simulink model "q_heli_2d_ff_lqr_i"  (Simulink 7.7)
settings: Solver=ode1  StartTime=0.0  StopTime=inf  FixedStep=0.002  MaxStep=10  RelTol=1e-3  AbsTol=1e-3
values from neighbouring files (symbols this model uses):
  g = 9.81    [setup_heli_2d_configuration.m]
  INT_JOYSTICK_SAT_LOWER = theta_0 * 180 / pi    (= -40.5)    [setup_lab_heli_2d.m]
  INT_JOYSTICK_SAT_UPPER = abs(theta_0)  * 180 / pi    [setup_lab_heli_2d.m]
  J_eq_p = J_m_p + J_body_p + J_p + J_y    (= 0.0384309870395)    [setup_heli_2d_configuration.m]
  J_eq_y = J_m_y + J_body_y + J_p + J_y + J_shaft    (= 0.0431517259335)    [setup_heli_2d_configuration.m]
  JOYSTICK_X_DZ = 0.25    [setup_lab_heli_2d.m]
  JOYSTICK_Y_DZ = 0.25    [setup_lab_heli_2d.m]
  K_AMP = 3    [setup_lab_heli_2d.m]
  K_EC_P = - 2 * pi / ( 4 * 1024 )    (= -0.00153398078789)    [setup_lab_heli_2d.m]
  K_EC_Y = 2 * pi / ( 8 * 1024 )    (= 0.000766990393943)    [setup_lab_heli_2d.m]
  K_ff = 1    [setup_lab_heli_2d.m]
  K_JOYSTICK_X = 85    [setup_lab_heli_2d.m]
  K_JOYSTICK_Y = 85    [setup_lab_heli_2d.m]
  K_pp = K_f_p * r_p    (= 0.20413345)    [setup_heli_2d_configuration.m]
  K_py = K_t_y / R_m_y    (= 0.0068125)    [setup_heli_2d_configuration.m]
  K_yp = K_t_p / R_m_p    (= 0.0219277108434)    [setup_heli_2d_configuration.m]
  K_yy = K_f_y * r_y    (= 0.071988045)    [setup_heli_2d_configuration.m]
  l_cm = ( (m_motor_p + m_shield ) * r_p +  (m_motor_y + m_shield ) * r_y ) / ( m_props )    (= 0.185670125995)    [setup_heli_2d_configuration.m]
  m_heli = 1.3872    [setup_heli_2d_configuration.m]
  SAT_INT_ERR_PITCH = 8    [setup_lab_heli_2d.m]
  SAT_INT_ERR_YAW = 8    [setup_lab_heli_2d.m]
  theta_0 = -40.5*pi/180    (= -0.706858347058)    [setup_lab_heli_2d.m]
  Tr_p = 1    [setup_lab_heli_2d.m]
  Tr_y = 1    [setup_lab_heli_2d.m]
  VMAX_AMP_P = 24    [setup_lab_heli_2d.m]
  VMAX_AMP_Y = 15    [setup_lab_heli_2d.m]
  wcf = 2 * pi * 20    (= 125.663706144)    [setup_lab_heli_2d.m]
  zetaf = 0.85    [setup_lab_heli_2d.m]
undefined symbols (not defined in the file or in its folder): B_p, B_y, HIL, K, Ki, qc_get_step_size
libraries: simulink x9, simulink_extras x7, quarc_library x4
settings Model: Creator=MLevis  LastModifiedBy=pmartin  SimulationMode=external  ExtModeTrigDuration=50000  BufferReuse=off
settings SolverCC: PositivePriorityOrder=on
settings DataIOCC: LimitDataPoints=off  SaveOutput=off  SaveTime=off  SignalLoggingName=sigsOut
settings OptimizationCC: BlockReduction=off  BooleanDataType=off  InlineInvariantSignals=on  OptimizeBlockIOStorage=off  BufferReuse=off  ExpressionFolding=off  LocalBlockOutputs=off  InitFltsAndDblsToZero=on
settings DebuggingCC: SaveWithParameterizedLinksMsg=none  SignalResolutionControl=TryResolveAllWithWarning  SolverPrmCheckMsg=none  MultiTaskDSMMsg=warning  MultiTaskCondExecSysMsg=none  StrictBusMsg=None
settings RTWCC: SystemTargetFile=quarc_windows.tlc  TemplateMakefile=quarc_default_tmf  Description=QuaRC Win32 Target  ProcessScript=quarc_windows_make_rtw_hook  IncludeERTFirstTime=on
settings STFCustomTargetCC: TargetFcnLib=ansi_tfl_tmw.mat  TargetPreCompLibLocation=C:\PROGRA~3\QUARC\lib\2012b\windows\release  GeneratePreprocessorConditionals=Disable all  SystemTargetFile=quarc_windows.tlc
settings GRTTargetCC: TargetFcnLib=ansi_tfl_tmw.mat  TargetPreCompLibLocation=C:\PROGRA~3\QUARC\lib\2012b\windows\release  ParMdlRefBuildCompliant=off  CompOptLevelCompliant=off  MatFileLogging=off  ExtMode=on  ExtModeMexFile=quarc_comm

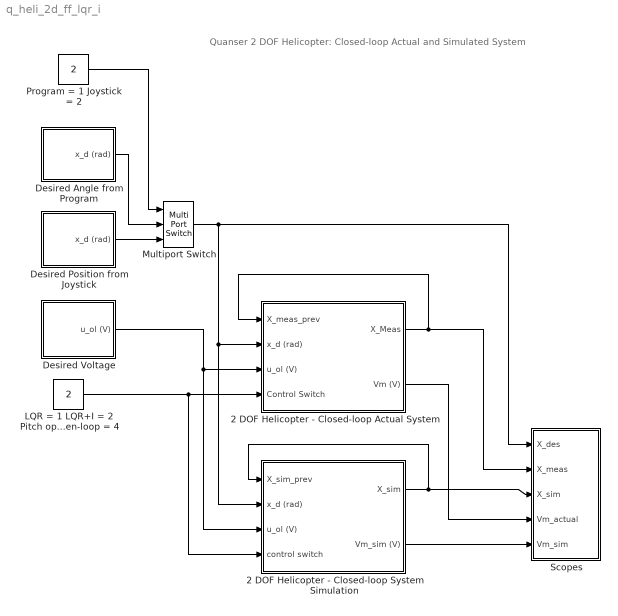
== system q_heli_2d_ff_lqr_i ==
  note: Quanser 2 DOF Helicopter:
      | Closed-loop Actual and Simulated System
  2 DOF Helicopter - Closed-loop Actual System : Subsystem
  2 DOF Helicopter - Closed-loop System Simulation : Subsystem
  Desired Angle from Program : Subsystem
  Desired Position from Joystick : Subsystem
  Desired Voltage : Subsystem
  LQR = 1 LQR+I = 2 Pitch open-loop  = 3 Yaw open-loop = 4 : Constant  Value=2
  Multiport Switch : MultiPortSwitch  Inputs=2
  Program = 1 Joystick = 2 : Constant  Value=2
  Scopes : Subsystem
  wires:
  2 DOF Helicopter - Closed-loop System Simulation/1(X_sim) -> Scopes/3(X_sim), 2 DOF Helicopter - Closed-loop System Simulation/1(X_sim_prev)
  2 DOF Helicopter - Closed-loop Actual System/1(X_Meas) -> Scopes/2(X_meas), 2 DOF Helicopter - Closed-loop Actual System/1(X_meas_prev)
  2 DOF Helicopter - Closed-loop Actual System/2(Vm (V)) -> Scopes/4(Vm_actual)
  LQR = 1 LQR+I = 2 Pitch open-loop  = 3 Yaw open-loop = 4/1 -> 2 DOF Helicopter - Closed-loop Actual System/4(Control Switch), 2 DOF Helicopter - Closed-loop System Simulation/4(control switch)
  2 DOF Helicopter - Closed-loop System Simulation/2(Vm_sim (V)) -> Scopes/5(Vm_sim)
  Desired Voltage/1(u_ol (V)) -> 2 DOF Helicopter - Closed-loop Actual System/3(u_ol (V)), 2 DOF Helicopter - Closed-loop System Simulation/3(u_ol (V))
  Program = 1 Joystick = 2/1 -> Multiport Switch/1
  Desired Angle from Program/1(x_d (rad)) -> Multiport Switch/2
  Desired Position from Joystick/1(x_d (rad)) -> Multiport Switch/3
  Multiport Switch/1 -> Scopes/1(X_des), 2 DOF Helicopter - Closed-loop Actual System/2(x_d (rad)), 2 DOF Helicopter - Closed-loop System Simulation/2(x_d (rad))

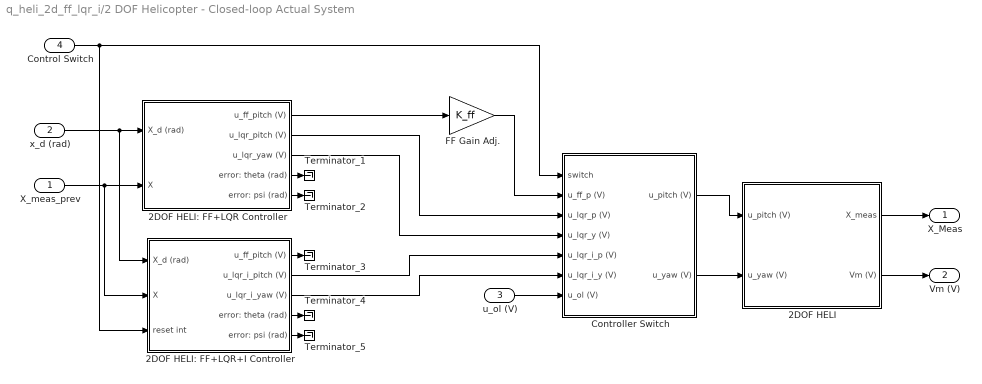
== system q_heli_2d_ff_lqr_i/2 DOF Helicopter - Closed-loop Actual System ==
  X_meas_prev : Inport
  x_d (rad) : Inport  Port=2
  u_ol (V) : Inport  Port=3
  Control Switch : Inport  Port=4
  2DOF HELI : Subsystem
  2DOF HELI: FF+LQR Controller : Subsystem
  2DOF HELI: FF+LQR+I Controller : Subsystem
  Controller Switch : Subsystem
  FF Gain Adj. : Gain  Gain=K_ff
  Terminator_{1..5} (5 alike) : Terminator
  X_Meas : Outport
  Vm (V) : Outport  Port=2
  wires:
  2DOF HELI: FF+LQR+I Controller/5(error: psi (rad)) -> Terminator_5/1
  2DOF HELI: FF+LQR+I Controller/4(error: theta (rad)) -> Terminator_4/1
  2DOF HELI: FF+LQR+I Controller/1(u_ff_pitch (V)) -> Terminator_3/1
  2DOF HELI: FF+LQR Controller/5(error: psi (rad)) -> Terminator_2/1
  2DOF HELI: FF+LQR Controller/4(error: theta (rad)) -> Terminator_1/1
  u_ol (V)/1 -> Controller Switch/7(u_ol (V))
  2DOF HELI: FF+LQR+I Controller/3(u_lqr_i_yaw (V)) -> Controller Switch/6(u_lqr_i_y (V))
  2DOF HELI: FF+LQR+I Controller/2(u_lqr_i_pitch (V)) -> Controller Switch/5(u_lqr_i_p (V))
  Controller Switch/2(u_yaw (V)) -> 2DOF HELI/2(u_yaw (V))
  Controller Switch/1(u_pitch (V)) -> 2DOF HELI/1(u_pitch (V))
  2DOF HELI: FF+LQR Controller/2(u_lqr_pitch (V)) -> Controller Switch/3(u_lqr_p (V))
  FF Gain Adj./1 -> Controller Switch/2(u_ff_p (V))
  2DOF HELI: FF+LQR Controller/3(u_lqr_yaw (V)) -> Controller Switch/4(u_lqr_y (V))
  X_meas_prev/1 -> 2DOF HELI: FF+LQR+I Controller/2(X), 2DOF HELI: FF+LQR Controller/2(X)
  x_d (rad)/1 -> 2DOF HELI: FF+LQR+I Controller/1(X_d (rad)), 2DOF HELI: FF+LQR Controller/1(X_d (rad))
  2DOF HELI: FF+LQR Controller/1(u_ff_pitch (V)) -> FF Gain Adj./1
  Control Switch/1 -> Controller Switch/1(switch), 2DOF HELI: FF+LQR+I Controller/3(reset int)
  2DOF HELI/2(Vm (V)) -> Vm (V)/1
  2DOF HELI/1(X_meas) -> X_Meas/1

== system q_heli_2d_ff_lqr_i/2 DOF Helicopter - Closed-loop System Simulation ==
  X_sim_prev : Inport
  x_d (rad) : Inport  Port=2
  u_ol (V) : Inport  Port=3
  control switch : Inport  Port=4
  2DOF HELI: FF+LQR Controller : Subsystem
  2DOF HELI: FF+LQR+I Controller : Subsystem
  2DOF HELI: Nonlinear Model : Subsystem
  Controller Switch : Subsystem
  Terminator_{1..5} (5 alike) : Terminator
  X_sim : Outport
  Vm_sim (V) : Outport  Port=2
  wires:
  2DOF HELI: FF+LQR+I Controller/5(error: psi (rad)) -> Terminator_5/1
  2DOF HELI: FF+LQR+I Controller/4(error: theta (rad)) -> Terminator_4/1
  2DOF HELI: FF+LQR+I Controller/1(u_ff_pitch (V)) -> Terminator_3/1
  2DOF HELI: FF+LQR Controller/5(error: psi (rad)) -> Terminator_2/1
  2DOF HELI: FF+LQR Controller/4(error: theta (rad)) -> Terminator_1/1
  u_ol (V)/1 -> Controller Switch/7(u_ol (V))
  2DOF HELI: Nonlinear Model/1(X_sim) -> X_sim/1
  2DOF HELI: Nonlinear Model/2(V_m_sim (V)) -> Vm_sim (V)/1
  control switch/1 -> 2DOF HELI: FF+LQR+I Controller/3(reset int), Controller Switch/1(switch)
  2DOF HELI: FF+LQR+I Controller/2(u_lqr_i_pitch (V)) -> Controller Switch/5(u_lqr_i_p (V))
  2DOF HELI: FF+LQR Controller/3(u_lqr_yaw (V)) -> Controller Switch/4(u_lqr_y (V))
  2DOF HELI: FF+LQR Controller/1(u_ff_pitch (V)) -> Controller Switch/2(u_ff_p (V))
  2DOF HELI: FF+LQR Controller/2(u_lqr_pitch (V)) -> Controller Switch/3(u_lqr_p (V))
  2DOF HELI: FF+LQR+I Controller/3(u_lqr_i_yaw (V)) -> Controller Switch/6(u_lqr_i_y (V))
  X_sim_prev/1 -> 2DOF HELI: FF+LQR+I Controller/2(X), 2DOF HELI: FF+LQR Controller/2(X)
  x_d (rad)/1 -> 2DOF HELI: FF+LQR Controller/1(X_d (rad)), 2DOF HELI: FF+LQR+I Controller/1(X_d (rad))
  Controller Switch/1(u_pitch (V)) -> 2DOF HELI: Nonlinear Model/1(u_pitch (V))
  Controller Switch/2(u_yaw (V)) -> 2DOF HELI: Nonlinear Model/2(u_yaw (V))

== system q_heli_2d_ff_lqr_i/Desired Angle from Program ==
  note: Desired yaw angle
  note: Desired pitch angle
  Amplitude: Pitch (deg) : Gain  Gain=0
  Amplitude: Yaw (deg) : Gain  Gain=0
  Constant : Constant
  Constant: Pitch (deg) : simulink/Math Operations/Slider Gain  low=-30  gain=-30  high=15
  Constant: Yaw (deg) : Constant  Value=0
  Mux : Mux  Inputs=2
  Pitch: deg to rad : simulink_extras/Transformations/Degrees to Radians
  Signal Generator: Pitch : SignalGenerator  WaveForm=square  Frequency=0.05
  Signal Generator: Yaw : SignalGenerator  WaveForm=square  Frequency=0.05
  Sum : Sum  Inputs=|++
  Sum1 : Sum  Inputs=|++
  Yaw: deg to rad : simulink_extras/Transformations/Degrees to Radians
  x_d (rad) : Outport
  wires:
  Constant: Pitch (deg)/1 -> Sum/2
  Yaw: deg to rad/1 -> Mux/2
  Mux/1 -> x_d (rad)/1
  Constant: Yaw (deg)/1 -> Sum1/2
  Amplitude: Yaw (deg)/1 -> Sum1/1
  Signal Generator: Yaw/1 -> Amplitude: Yaw (deg)/1
  Sum1/1 -> Yaw: deg to rad/1
  Constant/1 -> Constant: Pitch (deg)/1
  Amplitude: Pitch (deg)/1 -> Sum/1
  Signal Generator: Pitch/1 -> Amplitude: Pitch (deg)/1
  Sum/1 -> Pitch: deg to rad/1
  Pitch: deg to rad/1 -> Mux/1

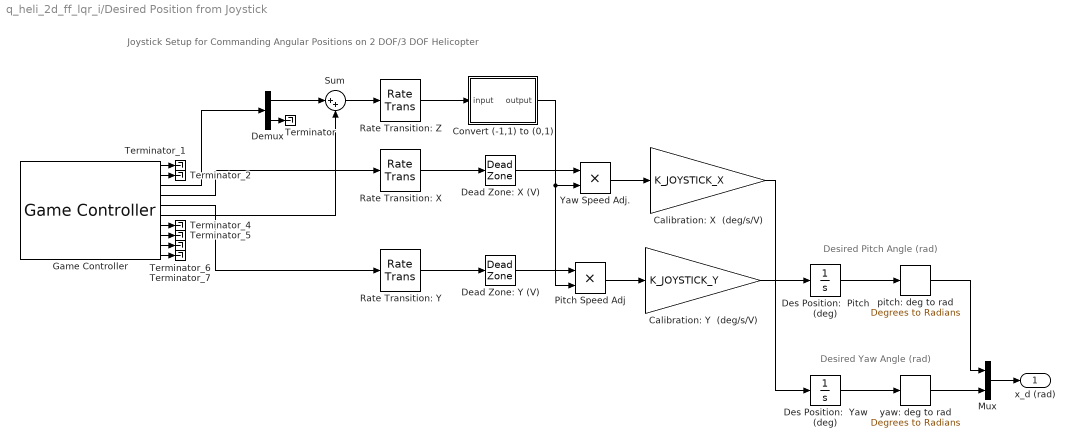
== system q_heli_2d_ff_lqr_i/Desired Position from Joystick ==
  note: Desired Pitch Angle (rad)
  note: Desired Yaw Angle (rad)
  note: Joystick Setup for Commanding Angular Positions on 2 DOF/3 DOF Helicopter
  Calibration: X  (deg/s/V) : Gain  Gain=K_JOYSTICK_X
  Calibration: Y  (deg/s/V) : Gain  Gain=K_JOYSTICK_Y
  Convert (-1,1) to (0,1) : Subsystem
  Dead Zone: X (V) : DeadZone  LowerValue=-JOYSTICK_X_DZ  UpperValue=JOYSTICK_X_DZ  SaturateOnIntegerOverflow=on
  Dead Zone: Y (V) : DeadZone  LowerValue=-JOYSTICK_Y_DZ  UpperValue=JOYSTICK_Y_DZ  SaturateOnIntegerOverflow=on
  Demux : Demux  Outputs=2
  Des Position:  Pitch (deg) : Integrator  InitialCondition=theta_0*180/pi  LimitOutput=on  UpperSaturationLimit=INT_JOYSTICK_SAT_UPPER  LowerSaturationLimit=INT_JOYSTICK_SAT_LOWER
  Des Position:  Yaw (deg) : Integrator  UpperSaturationLimit=180  LowerSaturationLimit=-180
  Game Controller : quarc_library/Devices/Peripherals/Target/Game Controller  controller=1  buffer_size=12  deadzone=[]  saturation=[]  sample_time=max(qc_get_step_size, 0.01)  auto_center=off  enabled=on
  Mux : Mux  Inputs=2
  Pitch Speed Adj : Product  RndMeth=Zero
  Rate Transition: X : RateTransition
  Rate Transition: Y : RateTransition
  Rate Transition: Z : RateTransition
  Sum : Sum  Inputs=|++
  Terminator : Terminator
  Terminator_{1..2,4..7} (6 alike) : Terminator
  Yaw Speed Adj. : Product  RndMeth=Zero
  pitch: deg to rad : simulink_extras/Transformations/Degrees to Radians
  yaw: deg to rad : simulink_extras/Transformations/Degrees to Radians
  x_d (rad) : Outport
  wires:
  Des Position:  Pitch (deg)/1 -> pitch: deg to rad/1
  Des Position:  Yaw (deg)/1 -> yaw: deg to rad/1
  Mux/1 -> x_d (rad)/1
  Calibration: X  (deg/s/V)/1 -> Des Position:  Yaw (deg)/1
  Dead Zone: X (V)/1 -> Yaw Speed Adj./1
  Dead Zone: Y (V)/1 -> Pitch Speed Adj/1
  pitch: deg to rad/1 -> Mux/1
  yaw: deg to rad/1 -> Mux/2
  Yaw Speed Adj./1 -> Calibration: X  (deg/s/V)/1
  Pitch Speed Adj/1 -> Calibration: Y  (deg/s/V)/1
  Calibration: Y  (deg/s/V)/1 -> Des Position:  Pitch (deg)/1
  Convert (-1,1) to (0,1)/1(output) -> Yaw Speed Adj./2, Pitch Speed Adj/2
  Rate Transition: X/1 -> Dead Zone: X (V)/1
  Rate Transition: Y/1 -> Dead Zone: Y (V)/1
  Rate Transition: Z/1 -> Convert (-1,1) to (0,1)/1(input)
  Game Controller/4 -> Rate Transition: X/1
  Game Controller/5 -> Rate Transition: Y/1
  Game Controller/1 -> Terminator_1/1
  Game Controller/2 -> Terminator_2/1
  Game Controller/7 -> Terminator_4/1
  Game Controller/8 -> Terminator_5/1
  Game Controller/9 -> Terminator_6/1
  Game Controller/10 -> Terminator_7/1
  Sum/1 -> Rate Transition: Z/1
  Game Controller/6 -> Sum/2
  Game Controller/3 -> Demux/1
  Demux/1 -> Sum/1
  Demux/2 -> Terminator/1

== system q_heli_2d_ff_lqr_i/Desired Voltage ==
  note: Desired pitch open-loop voltage
  note: Desired yaw open-loop voltage
  Amplitude: Pitch (V) : Gain  Gain=0.2
  Amplitude: Yaw (V) : Gain  Gain=2.5
  Constant: Pitch (V) : Constant  Value=0
  Constant: Yaw (V) : Constant  Value=0
  Mux : Mux  Inputs=2
  Signal Generator: Pitch (V) : SignalGenerator  WaveForm=square  Frequency=0.4
  Signal Generator: Yaw (V) : SignalGenerator  WaveForm=square  Frequency=0.01
  Sum : Sum  Inputs=|++
  Sum1 : Sum  Inputs=|++
  u_ol (V) : Outport
  wires:
  Constant: Pitch (V)/1 -> Sum/2
  Amplitude: Pitch (V)/1 -> Sum/1
  Signal Generator: Pitch (V)/1 -> Amplitude: Pitch (V)/1
  Constant: Yaw (V)/1 -> Sum1/2
  Amplitude: Yaw (V)/1 -> Sum1/1
  Signal Generator: Yaw (V)/1 -> Amplitude: Yaw (V)/1
  Sum/1 -> Mux/1
  Sum1/1 -> Mux/2
  Mux/1 -> u_ol (V)/1

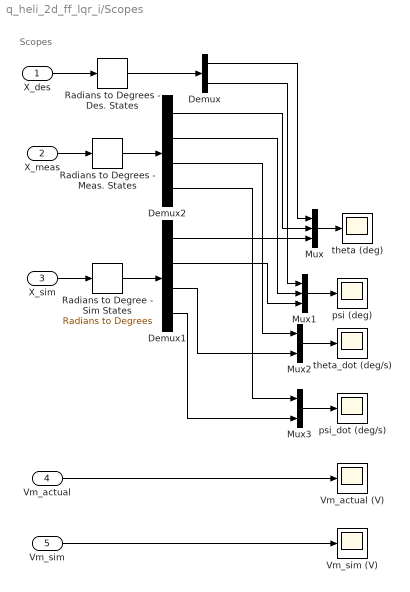
== system q_heli_2d_ff_lqr_i/Scopes ==
  note: Scopes
  X_des : Inport
  X_meas : Inport  Port=2
  X_sim : Inport  Port=3
  Vm_actual : Inport  Port=4
  Vm_sim : Inport  Port=5
  Demux : Demux  Outputs=2
  Demux1 : Demux
  Demux2 : Demux
  Mux : Mux  Inputs=3
  Mux1 : Mux  Inputs=3
  Mux2 : Mux  Inputs=2
  Mux3 : Mux  Inputs=2
  Radians to Degree - Sim States : simulink_extras/Transformations/Radians to Degrees
  Radians to Degrees - Des. States : simulink_extras/Transformations/Radians to Degrees
  Radians to Degrees - Meas. States : simulink_extras/Transformations/Radians to Degrees
  Vm_actual (V) : Scope
      settings: TickLabels=on  TimeRange=50  YMax=15  SaveName=ScopeData4
  Vm_sim (V) : Scope
      settings: TickLabels=on  TimeRange=1.000000  YMin=-250  YMax=250  SaveName=ScopeData5
  psi (deg) : Scope
      settings: TickLabels=on  TimeRange=50  YMin=-70  YMax=90
  psi_dot (deg/s) : Scope
      settings: TickLabels=on  TimeRange=1.000000  YMin=-250  YMax=250  SaveName=ScopeData3
  theta (deg) : Scope
      settings: TickLabels=on  TimeRange=50  YMin=-27.5  YMax=30
  theta_dot (deg/s) : Scope
      settings: TickLabels=on  TimeRange=1.000000  YMax=3.5  SaveName=ScopeData2
  wires:
  Vm_sim/1 -> Vm_sim (V)/1
  Radians to Degrees - Des. States/1 -> Demux/1
  Demux1/2 -> Mux1/3
  Demux2/2 -> Mux1/2
  Demux/2 -> Mux1/1
  Demux1/1 -> Mux/3
  Demux2/1 -> Mux/2
  Demux/1 -> Mux/1
  X_des/1 -> Radians to Degrees - Des. States/1
  Demux2/3 -> Mux2/1
  Demux2/4 -> Mux3/1
  X_meas/1 -> Radians to Degrees - Meas. States/1
  Radians to Degrees - Meas. States/1 -> Demux2/1
  X_sim/1 -> Radians to Degree - Sim States/1
  Radians to Degree - Sim States/1 -> Demux1/1
  Mux/1 -> theta (deg)/1
  Mux1/1 -> psi (deg)/1
  Mux2/1 -> theta_dot (deg/s)/1
  Mux3/1 -> psi_dot (deg/s)/1
  Demux1/3 -> Mux2/2
  Demux1/4 -> Mux3/2
  Vm_actual/1 -> Vm_actual (V)/1

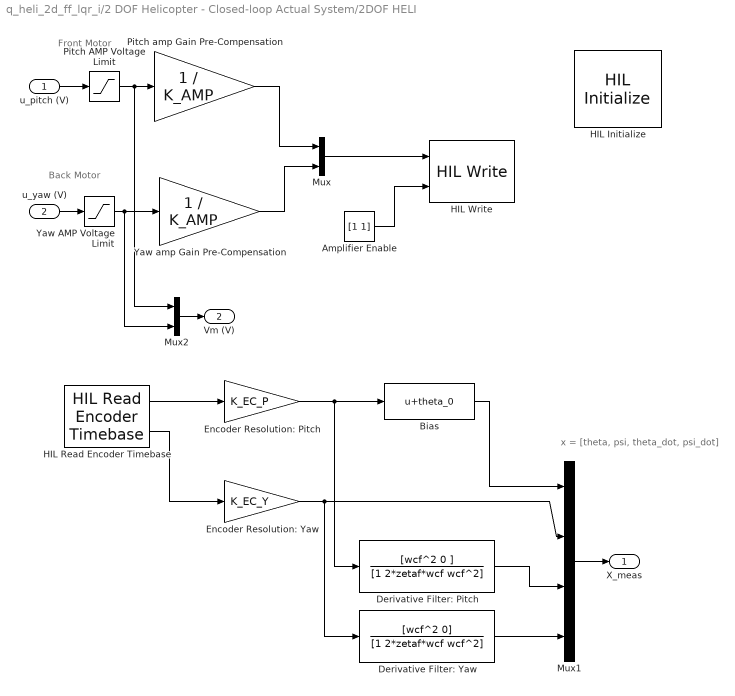
== system q_heli_2d_ff_lqr_i/2 DOF Helicopter - Closed-loop Actual System/2DOF HELI ==
  note: x = [theta, psi, theta_dot, psi_dot]
  note: Front Motor
  note: Back Motor
  u_pitch (V) : Inport
  u_yaw (V) : Inport  Port=2
  Amplifier Enable : Constant  Value=[1 1]
  Bias : Bias  Bias=theta_0
  Derivative Filter: Pitch : TransferFcn  Numerator=[wcf^2 0 ]  Denominator=[1 2*zetaf*wcf wcf^2]
  Derivative Filter: Yaw : TransferFcn  Numerator=[wcf^2 0]  Denominator=[1 2*zetaf*wcf wcf^2]
  "Encoder Resolution: Pitch " : Gain  Gain=K_EC_P
  Encoder Resolution: Yaw : Gain  Gain=K_EC_Y
  HIL Initialize : quarc_library/Data Acquisition/Generic/Configuration/HIL Initialize  object_name=HIL-1  board_type=q2_usb  board_number=0  board_options=d0=digital;d1=digital;led=auto;update_rate=normal;decimation=1  exclusive=off  active=on  hardware_clocks=[0]  clock_modes=[]  initial_clock_frequencies=[]  set_clock_params_at_start=off  set_clock_params_at_switch_in=off  set_clock_frequencies_at_start=off  set_clock_frequencies_at_switch_in=off  analog_input_channels=[0:1]  analog_input_maximums=10  analog_input_minimums=-10  set_analog_input_params_at_start=on  set_analog_input_params_at_switch_in=off  analog_output_channels=[0:1]  analog_output_maximums=10  analog_output_minimums=-10  initial_analog_outputs=[0]  final_analog_outputs=[0]  watchdog_analog_outputs=0  set_analog_output_params_at_start=on  set_analog_output_params_at_switch_in=off  set_analog_outputs_at_start=on  set_analog_outputs_at_switch_in=off  set_analog_outputs_at_terminate=on  set_analog_outputs_at_switch_out=off  set_analog_outputs_on_watchdog=off  digital_input_channels=[]  digital_output_channels=[0:1]  digital_output_configuration=[]  initial_digital_outputs=[0]  final_digital_outputs=[0]  watchdog_digital_outputs=[0]  set_digital_output_params_at_start=off  set_digital_output_params_at_switch_in=off  set_digital_outputs_at_start=on  set_digital_outputs_at_switch_in=off  set_digital_outputs_at_terminate=on  set_digital_outputs_at_switch_out=off  set_digital_outputs_on_watchdog=on  encoder_channels=[0:1]  quadrature=[4]  encoder_filter_frequency=[]  initial_encoder_counts=[0]  set_encoder_params_at_start=on  set_encoder_params_at_switch_in=off  set_encoder_counts_at_start=on  set_encoder_counts_at_switch_in=off  pwm_channels=[]  pwm_modes=[0]  pwm_frequency=1/0.020  pwm_configuration=[]  pwm_alignment=[]  pwm_polarity=[]  pwm_leading_deadband=[]  pwm_trailing_deadband=[]  initial_pwm_outputs=[0]  final_pwm_outputs=[0]  watchdog_pwm_outputs=[0]  set_pwm_params_at_start=on  set_pwm_params_at_switch_in=off  set_pwm_outputs_at_start=on  set_pwm_outputs_at_switch_in=off  set_pwm_outputs_at_terminate=on  set_pwm_outputs_at_switch_out=off  set_pwm_outputs_on_watchdog=off  other_output_channels=[]  initial_other_outputs=[]  final_other_outputs=[]  watchdog_other_outputs=[]  set_other_outputs_at_start=off  set_other_outputs_at_switch_in=off  set_other_outputs_at_terminate=off  set_other_outputs_at_switch_out=off  set_other_outputs_on_watchdog=off
  HIL Read Encoder Timebase : quarc_library/Data Acquisition/Generic/Timebases/HIL Read Encoder Timebase  object_name=HIL-1  clock=0  channels=[0:1]  samples_in_buffer=max(ceil(1/qc_get_step_size), 1)  active=on  vector_output=off  data_type_mode=Inherit via back propagation  data_type=double
  HIL Write : quarc_library/Data Acquisition/Generic/Immediate I//O/HIL Write  object_name=HIL-1  analog_channels=0:1  pwm_channels=[]  digital_channels=0:1  other_channels=[]  sample_time=-1  active=off  vector_input=on
  Mux : Mux  Inputs=2
  Mux1 : Mux
  Mux2 : Mux  Inputs=2
  Pitch AMP Voltage Limit : Saturate  UpperLimit=VMAX_AMP_P  LowerLimit=- VMAX_AMP_P
  Pitch amp Gain Pre-Compensation : Gain  Gain=1 / K_AMP  SaturateOnIntegerOverflow=on  OutDataTypeStr=Inherit: Same as input  ParamDataTypeStr=Inherit: Same as input
  Yaw AMP Voltage Limit : Saturate  UpperLimit=VMAX_AMP_Y  LowerLimit=- VMAX_AMP_Y
  Yaw amp Gain Pre-Compensation : Gain  Gain=1 / K_AMP  SaturateOnIntegerOverflow=on  OutDataTypeStr=Inherit: Same as input  ParamDataTypeStr=Inherit: Same as input
  X_meas : Outport
  Vm (V) : Outport  Port=2
  wires:
  Derivative Filter: Yaw/1 -> Mux1/4
  Derivative Filter: Pitch/1 -> Mux1/3
  Bias/1 -> Mux1/1
  HIL Read Encoder Timebase/2 -> Encoder Resolution: Yaw/1
  "Encoder Resolution: Pitch "/1 -> Derivative Filter: Pitch/1, Bias/1
  HIL Read Encoder Timebase/1 -> "Encoder Resolution: Pitch "/1
  Mux/1 -> HIL Write/1
  Pitch AMP Voltage Limit/1 -> Pitch amp Gain Pre-Compensation/1, Mux2/1
  Yaw AMP Voltage Limit/1 -> Yaw amp Gain Pre-Compensation/1, Mux2/2
  u_pitch (V)/1 -> Pitch AMP Voltage Limit/1
  u_yaw (V)/1 -> Yaw AMP Voltage Limit/1
  Mux1/1 -> X_meas/1
  Pitch amp Gain Pre-Compensation/1 -> Mux/1
  Yaw amp Gain Pre-Compensation/1 -> Mux/2
  Mux2/1 -> Vm (V)/1
  Encoder Resolution: Yaw/1 -> Derivative Filter: Yaw/1, Mux1/2
  Amplifier Enable/1 -> HIL Write/2

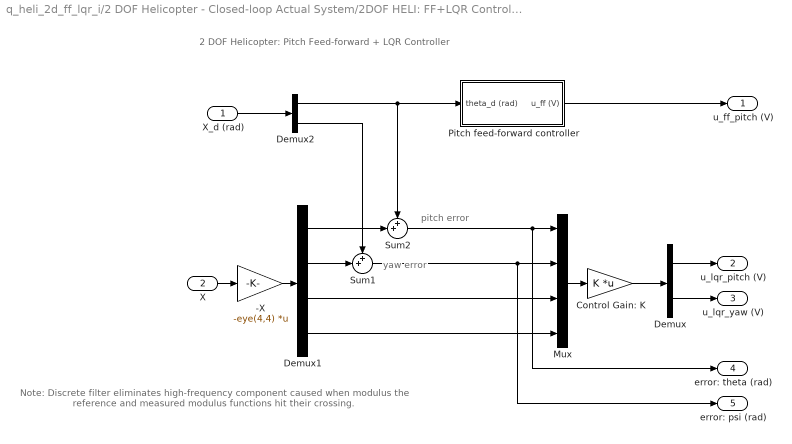
== system q_heli_2d_ff_lqr_i/2 DOF Helicopter - Closed-loop Actual System/2DOF HELI: FF+LQR Controller ==
  note: yaw error
  note: pitch error
  note: 2 DOF Helicopter:
      | Pitch Feed-forward + LQR Controller
  note: Note: Discrete filter eliminates high-frequency
      | component caused when modulus the reference
      | and measured modulus functions hit their crossing.
  X_d (rad) : Inport
  X : Inport  Port=2
  -X : Gain  Gain=-eye(4,4)  Multiplication=Matrix(K*u)
  Control Gain: K : Gain  Gain=K  Multiplication=Matrix(K*u)
  Demux : Demux  Outputs=2
  Demux1 : Demux
  Demux2 : Demux  Outputs=2
  Mux : Mux
  Pitch feed-forward controller : Subsystem
  Sum1 : Sum  Inputs=++|
  Sum2 : Sum  Inputs=++|
  u_ff_pitch (V) : Outport
  u_lqr_pitch (V) : Outport  Port=2
  u_lqr_yaw (V) : Outport  Port=3
  error: theta (rad) : Outport  Port=4
  error: psi (rad) : Outport  Port=5
  wires:
  Pitch feed-forward controller/1(u_ff (V)) -> u_ff_pitch (V)/1
  Demux/1 -> u_lqr_pitch (V)/1
  Demux/2 -> u_lqr_yaw (V)/1
  Sum2/1 -> Mux/1, error: theta (rad)/1
  Demux1/1 -> Sum2/2
  X/1 -> -X/1
  -X/1 -> Demux1/1
  Control Gain: K/1 -> Demux/1
  Mux/1 -> Control Gain: K/1
  Demux1/3 -> Mux/3
  Demux1/4 -> Mux/4
  X_d (rad)/1 -> Demux2/1
  Demux1/2 -> Sum1/2
  Demux2/2 -> Sum1/1
  Demux2/1 -> Pitch feed-forward controller/1(theta_d (rad)), Sum2/1
  Sum1/1 -> Mux/2, error: psi (rad)/1

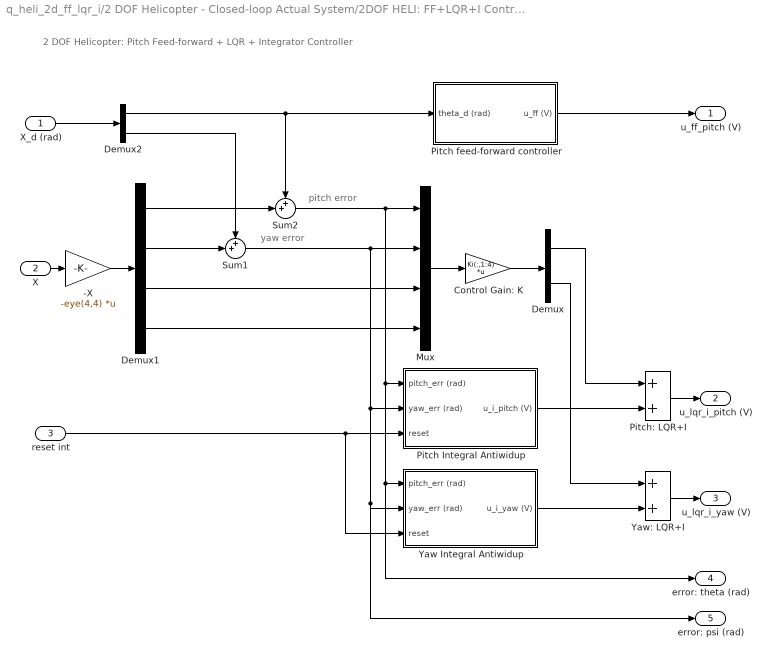
== system q_heli_2d_ff_lqr_i/2 DOF Helicopter - Closed-loop Actual System/2DOF HELI: FF+LQR+I Controller ==
  note: 2 DOF Helicopter:
      | Pitch Feed-forward + LQR + Integrator Controller
  note: pitch error
  note: yaw error
  X_d (rad) : Inport
  X : Inport  Port=2
  reset int : Inport  Port=3
  -X : Gain  Gain=-eye(4,4)  Multiplication=Matrix(K*u)
  Control Gain: K : Gain  Gain=Ki(:,1:4)  Multiplication=Matrix(K*u)
  Demux : Demux  Outputs=2
  Demux1 : Demux
  Demux2 : Demux  Outputs=2
  Mux : Mux
  Pitch Integral Antiwidup : Subsystem
  Pitch feed-forward controller : Subsystem
  Pitch: LQR+I : Sum
  Sum1 : Sum  Inputs=++|
  Sum2 : Sum  Inputs=++|
  Yaw Integral Antiwidup : Subsystem
  Yaw: LQR+I : Sum
  u_ff_pitch (V) : Outport
  u_lqr_i_pitch (V) : Outport  Port=2
  u_lqr_i_yaw (V) : Outport  Port=3
  error: theta (rad) : Outport  Port=4
  error: psi (rad) : Outport  Port=5
  wires:
  Demux1/4 -> Mux/4
  Demux1/3 -> Mux/3
  Mux/1 -> Control Gain: K/1
  Control Gain: K/1 -> Demux/1
  -X/1 -> Demux1/1
  Sum1/1 -> Mux/2, Pitch Integral Antiwidup/2(yaw_err (rad)), error: psi (rad)/1, Yaw Integral Antiwidup/2(yaw_err (rad))
  X/1 -> -X/1
  Demux1/1 -> Sum2/2
  Sum2/1 -> Pitch Integral Antiwidup/1(pitch_err (rad)), error: theta (rad)/1, Yaw Integral Antiwidup/1(pitch_err (rad)), Mux/1
  Pitch feed-forward controller/1(u_ff (V)) -> u_ff_pitch (V)/1
  Pitch Integral Antiwidup/1(u_i_pitch (V)) -> Pitch: LQR+I/2
  Demux/1 -> Pitch: LQR+I/1
  Pitch: LQR+I/1 -> u_lqr_i_pitch (V)/1
  Yaw: LQR+I/1 -> u_lqr_i_yaw (V)/1
  Demux/2 -> Yaw: LQR+I/1
  Yaw Integral Antiwidup/1(u_i_yaw (V)) -> Yaw: LQR+I/2
  X_d (rad)/1 -> Demux2/1
  Demux2/1 -> Pitch feed-forward controller/1(theta_d (rad)), Sum2/1
  Demux2/2 -> Sum1/1
  Demux1/2 -> Sum1/2
  reset int/1 -> Yaw Integral Antiwidup/3(reset), Pitch Integral Antiwidup/3(reset)

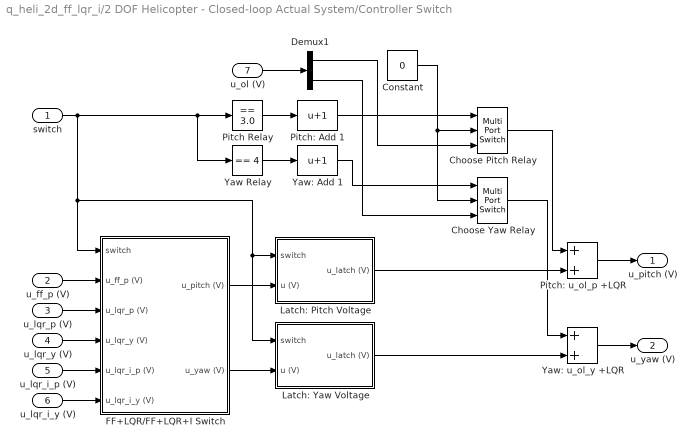
== system q_heli_2d_ff_lqr_i/2 DOF Helicopter - Closed-loop Actual System/Controller Switch ==
  switch : Inport
  u_ff_p (V) : Inport  Port=2
  u_lqr_p (V) : Inport  Port=3
  u_lqr_y (V) : Inport  Port=4
  u_lqr_i_p (V) : Inport  Port=5
  u_lqr_i_y (V) : Inport  Port=6
  u_ol (V) : Inport  Port=7
  Choose Pitch Relay : MultiPortSwitch  Inputs=2
  Choose Yaw Relay : MultiPortSwitch  Inputs=2
  Constant : Constant  Value=0
  Demux1 : Demux  Outputs=2
  FF+LQR/FF+LQR+I Switch : Subsystem
  Latch: Pitch Voltage : Subsystem
  Latch: Yaw Voltage : Subsystem
  Pitch Relay : simulink/Logic and Bit Operations/Compare To Constant  relop===  const=3.0  LogicOutDataTypeMode=uint8  ZeroCross=off
  Pitch: u_ol_p +LQR : Sum
  Pitch: Add 1 : Bias  Bias=1
  Yaw Relay : simulink/Logic and Bit Operations/Compare To Constant  relop===  const=4  LogicOutDataTypeMode=uint8  ZeroCross=off
  Yaw: u_ol_y +LQR : Sum
  Yaw: Add 1 : Bias  Bias=1
  u_pitch (V) : Outport
  u_yaw (V) : Outport  Port=2
  wires:
  FF+LQR/FF+LQR+I Switch/1(u_pitch (V)) -> Latch: Pitch Voltage/2(u (V))
  FF+LQR/FF+LQR+I Switch/2(u_yaw (V)) -> Latch: Yaw Voltage/2(u (V))
  u_ff_p (V)/1 -> FF+LQR/FF+LQR+I Switch/2(u_ff_p (V))
  u_lqr_p (V)/1 -> FF+LQR/FF+LQR+I Switch/3(u_lqr_p (V))
  u_lqr_y (V)/1 -> FF+LQR/FF+LQR+I Switch/4(u_lqr_y (V))
  u_lqr_i_p (V)/1 -> FF+LQR/FF+LQR+I Switch/5(u_lqr_i_p (V))
  u_lqr_i_y (V)/1 -> FF+LQR/FF+LQR+I Switch/6(u_lqr_i_y (V))
  Latch: Pitch Voltage/1(u_latch (V)) -> Pitch: u_ol_p +LQR/2
  Latch: Yaw Voltage/1(u_latch (V)) -> Yaw: u_ol_y +LQR/2
  switch/1 -> FF+LQR/FF+LQR+I Switch/1(switch), Latch: Pitch Voltage/1(switch), Latch: Yaw Voltage/1(switch), Pitch Relay/1, Yaw Relay/1
  Pitch: u_ol_p +LQR/1 -> u_pitch (V)/1
  Yaw: u_ol_y +LQR/1 -> u_yaw (V)/1
  Pitch Relay/1 -> Pitch: Add 1/1
  Pitch: Add 1/1 -> Choose Pitch Relay/1
  u_ol (V)/1 -> Demux1/1
  Yaw Relay/1 -> Yaw: Add 1/1
  Yaw: Add 1/1 -> Choose Yaw Relay/1
  Constant/1 -> Choose Pitch Relay/2, Choose Yaw Relay/2
  Demux1/1 -> Choose Pitch Relay/3
  Demux1/2 -> Choose Yaw Relay/3
  Choose Yaw Relay/1 -> Yaw: u_ol_y +LQR/1
  Choose Pitch Relay/1 -> Pitch: u_ol_p +LQR/1

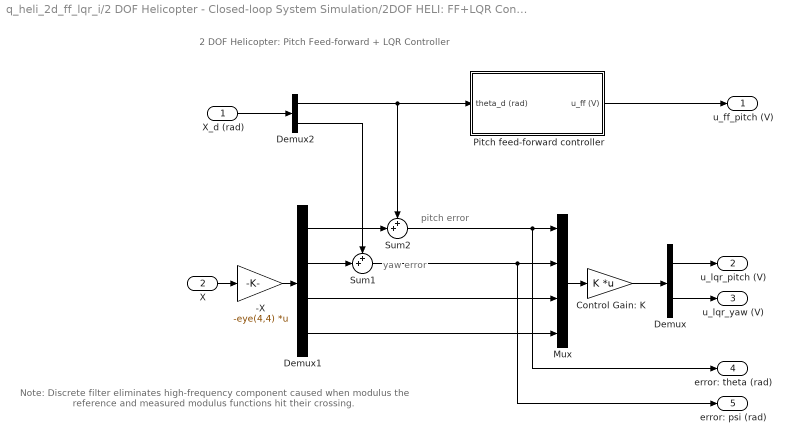
== system q_heli_2d_ff_lqr_i/2 DOF Helicopter - Closed-loop System Simulation/2DOF HELI: FF+LQR Controller ==
  note: yaw error
  note: pitch error
  note: 2 DOF Helicopter:
      | Pitch Feed-forward + LQR Controller
  note: Note: Discrete filter eliminates high-frequency
      | component caused when modulus the reference
      | and measured modulus functions hit their crossing.
  X_d (rad) : Inport
  X : Inport  Port=2
  -X : Gain  Gain=-eye(4,4)  Multiplication=Matrix(K*u)
  Control Gain: K : Gain  Gain=K  Multiplication=Matrix(K*u)
  Demux : Demux  Outputs=2
  Demux1 : Demux
  Demux2 : Demux  Outputs=2
  Mux : Mux
  Pitch feed-forward controller : Subsystem
  Sum1 : Sum  Inputs=++|
  Sum2 : Sum  Inputs=++|
  u_ff_pitch (V) : Outport
  u_lqr_pitch (V) : Outport  Port=2
  u_lqr_yaw (V) : Outport  Port=3
  error: theta (rad) : Outport  Port=4
  error: psi (rad) : Outport  Port=5
  wires:
  Pitch feed-forward controller/1(u_ff (V)) -> u_ff_pitch (V)/1
  Demux/1 -> u_lqr_pitch (V)/1
  Demux/2 -> u_lqr_yaw (V)/1
  Sum2/1 -> Mux/1, error: theta (rad)/1
  Demux1/1 -> Sum2/2
  X/1 -> -X/1
  -X/1 -> Demux1/1
  Control Gain: K/1 -> Demux/1
  Mux/1 -> Control Gain: K/1
  Demux1/3 -> Mux/3
  Demux1/4 -> Mux/4
  X_d (rad)/1 -> Demux2/1
  Demux1/2 -> Sum1/2
  Demux2/2 -> Sum1/1
  Demux2/1 -> Sum2/1, Pitch feed-forward controller/1(theta_d (rad))
  Sum1/1 -> Mux/2, error: psi (rad)/1

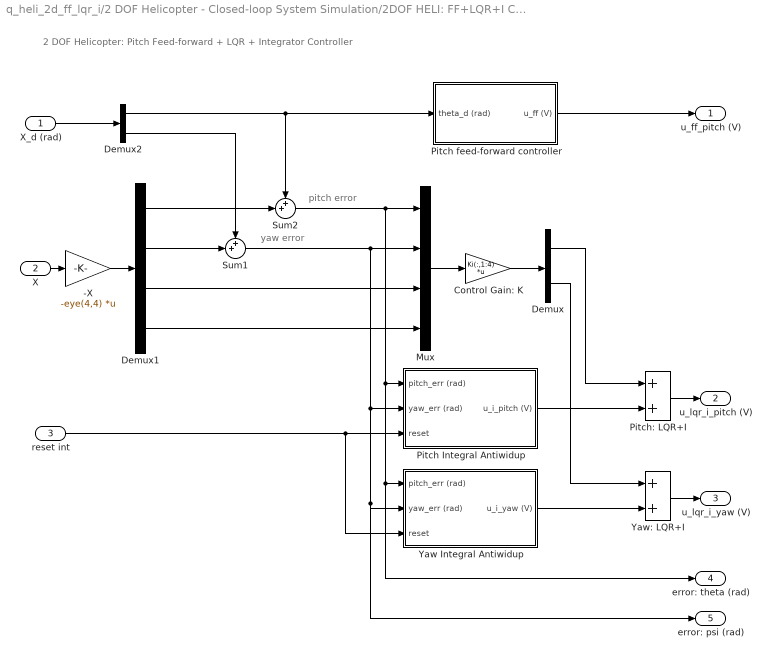
== system q_heli_2d_ff_lqr_i/2 DOF Helicopter - Closed-loop System Simulation/2DOF HELI: FF+LQR+I Controller ==
  note: 2 DOF Helicopter:
      | Pitch Feed-forward + LQR + Integrator Controller
  note: pitch error
  note: yaw error
  X_d (rad) : Inport
  X : Inport  Port=2
  reset int : Inport  Port=3
  -X : Gain  Gain=-eye(4,4)  Multiplication=Matrix(K*u)
  Control Gain: K : Gain  Gain=Ki(:,1:4)  Multiplication=Matrix(K*u)
  Demux : Demux  Outputs=2
  Demux1 : Demux
  Demux2 : Demux  Outputs=2
  Mux : Mux
  Pitch Integral Antiwidup : Subsystem
  Pitch feed-forward controller : Subsystem
  Pitch: LQR+I : Sum
  Sum1 : Sum  Inputs=++|
  Sum2 : Sum  Inputs=++|
  Yaw Integral Antiwidup : Subsystem
  Yaw: LQR+I : Sum
  u_ff_pitch (V) : Outport
  u_lqr_i_pitch (V) : Outport  Port=2
  u_lqr_i_yaw (V) : Outport  Port=3
  error: theta (rad) : Outport  Port=4
  error: psi (rad) : Outport  Port=5
  wires:
  Demux1/4 -> Mux/4
  Demux1/3 -> Mux/3
  Mux/1 -> Control Gain: K/1
  Control Gain: K/1 -> Demux/1
  -X/1 -> Demux1/1
  Sum1/1 -> Mux/2, Pitch Integral Antiwidup/2(yaw_err (rad)), error: psi (rad)/1, Yaw Integral Antiwidup/2(yaw_err (rad))
  X/1 -> -X/1
  Demux1/1 -> Sum2/2
  Sum2/1 -> Pitch Integral Antiwidup/1(pitch_err (rad)), error: theta (rad)/1, Yaw Integral Antiwidup/1(pitch_err (rad)), Mux/1
  Pitch feed-forward controller/1(u_ff (V)) -> u_ff_pitch (V)/1
  Pitch Integral Antiwidup/1(u_i_pitch (V)) -> Pitch: LQR+I/2
  Demux/1 -> Pitch: LQR+I/1
  Pitch: LQR+I/1 -> u_lqr_i_pitch (V)/1
  Yaw: LQR+I/1 -> u_lqr_i_yaw (V)/1
  Demux/2 -> Yaw: LQR+I/1
  Yaw Integral Antiwidup/1(u_i_yaw (V)) -> Yaw: LQR+I/2
  X_d (rad)/1 -> Demux2/1
  Demux2/1 -> Pitch feed-forward controller/1(theta_d (rad)), Sum2/1
  Demux2/2 -> Sum1/1
  Demux1/2 -> Sum1/2
  reset int/1 -> Yaw Integral Antiwidup/3(reset), Pitch Integral Antiwidup/3(reset)

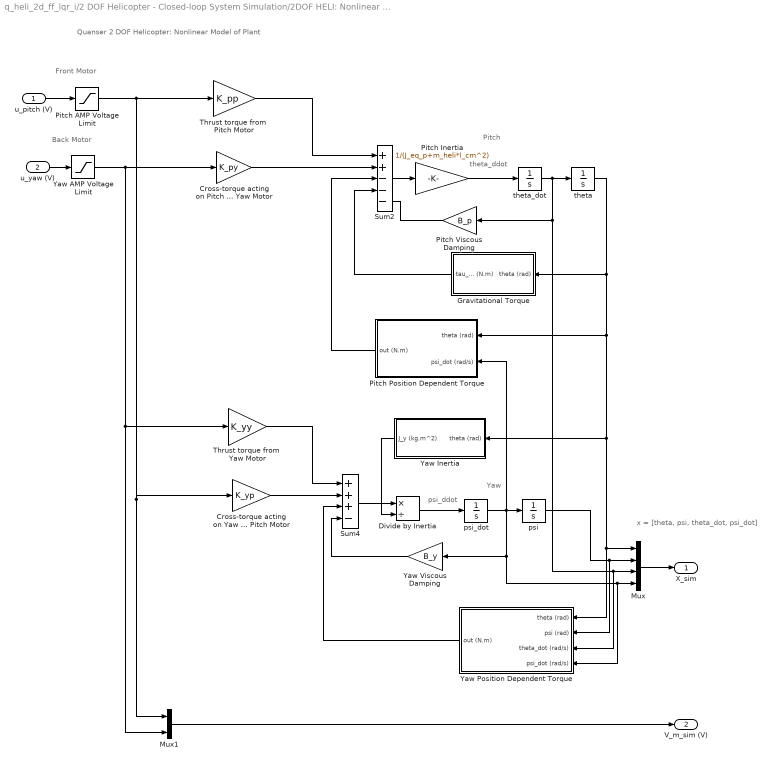
== system q_heli_2d_ff_lqr_i/2 DOF Helicopter - Closed-loop System Simulation/2DOF HELI: Nonlinear Model ==
  note: Yaw
  note: Pitch
  note: psi_ddot
  note: theta_ddot
  note: Quanser 2 DOF Helicopter: Nonlinear Model of Plant
  note: x = [theta, psi, theta_dot, psi_dot]
  note: Front Motor
  note: Back Motor
  u_pitch (V) : Inport
  u_yaw (V) : Inport  Port=2
  Cross-torque acting on Pitch  from Yaw Motor : Gain  Gain=K_py
  Cross-torque acting on Yaw  from Pitch Motor : Gain  Gain=K_yp
  Divide by Inertia : Product  Inputs=*/
  Gravitational Torque : Subsystem
  Mux : Mux
  Mux1 : Mux  Inputs=2
  Pitch AMP Voltage Limit : Saturate  UpperLimit=VMAX_AMP_P  LowerLimit=- VMAX_AMP_P
  Pitch Inertia : Gain  Gain=1/(J_eq_p+m_heli*l_cm^2)
  Pitch Position Dependent Torque : Subsystem
  Pitch Viscous Damping : Gain  Gain=B_p
  Sum2 : Sum  Inputs=++---
  Sum4 : Sum  Inputs=+++-
  Thrust torque from  Pitch Motor : Gain  Gain=K_pp
  Thrust torque from  Yaw Motor : Gain  Gain=K_yy
  Yaw AMP Voltage Limit : Saturate  UpperLimit=VMAX_AMP_Y  LowerLimit=- VMAX_AMP_Y
  Yaw Inertia : Subsystem
  Yaw Position Dependent Torque : Subsystem
  Yaw Viscous Damping : Gain  Gain=B_y
  psi : Integrator
  psi_dot : Integrator
  theta : Integrator  InitialCondition=theta_0  LimitOutput=on  UpperSaturationLimit=40.5*pi/180  LowerSaturationLimit=-40.5*pi/180
  theta_dot : Integrator
  X_sim : Outport
  V_m_sim (V) : Outport  Port=2
  wires:
  u_yaw (V)/1 -> Yaw AMP Voltage Limit/1
  u_pitch (V)/1 -> Pitch AMP Voltage Limit/1
  psi_dot/1 -> psi/1, Pitch Position Dependent Torque/2(psi_dot (rad/s)), Mux/4, Yaw Position Dependent Torque/4(psi_dot (rad/s)), Yaw Viscous Damping/1
  Cross-torque acting on Yaw  from Pitch Motor/1 -> Sum4/2
  Thrust torque from  Yaw Motor/1 -> Sum4/1
  theta_dot/1 -> theta/1, Mux/3, Yaw Position Dependent Torque/3(theta_dot (rad/s)), Pitch Viscous Damping/1
  Pitch Inertia/1 -> theta_dot/1
  Sum2/1 -> Pitch Inertia/1
  theta/1 -> Yaw Inertia/1(theta (rad)), Mux/1, Yaw Position Dependent Torque/1(theta (rad)), Pitch Position Dependent Torque/1(theta (rad)), Gravitational Torque/1(theta (rad))
  Mux/1 -> X_sim/1
  Pitch AMP Voltage Limit/1 -> Thrust torque from  Pitch Motor/1, Mux1/1, Cross-torque acting on Yaw  from Pitch Motor/1
  Yaw AMP Voltage Limit/1 -> Cross-torque acting on Pitch  from Yaw Motor/1, Mux1/2, Thrust torque from  Yaw Motor/1
  Mux1/1 -> V_m_sim (V)/1
  psi/1 -> Mux/2, Yaw Position Dependent Torque/2(psi (rad))
  Yaw Viscous Damping/1 -> Sum4/4
  Yaw Position Dependent Torque/1(out (N.m)) -> Sum4/3
  Sum4/1 -> Divide by Inertia/1
  Divide by Inertia/1 -> psi_dot/1
  Yaw Inertia/1(J_y (kg.m^2)) -> Divide by Inertia/2
  Thrust torque from  Pitch Motor/1 -> Sum2/1
  Cross-torque acting on Pitch  from Yaw Motor/1 -> Sum2/2
  Pitch Viscous Damping/1 -> Sum2/5
  Gravitational Torque/1(tau_g (N.m)) -> Sum2/4
  Pitch Position Dependent Torque/1(out (N.m)) -> Sum2/3

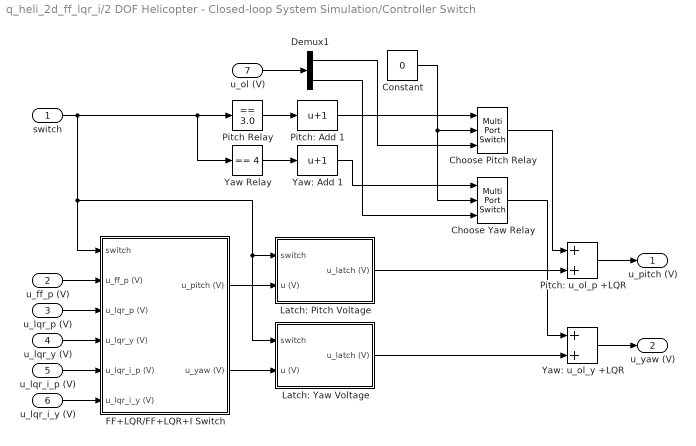
== system q_heli_2d_ff_lqr_i/2 DOF Helicopter - Closed-loop System Simulation/Controller Switch ==
  switch : Inport
  u_ff_p (V) : Inport  Port=2
  u_lqr_p (V) : Inport  Port=3
  u_lqr_y (V) : Inport  Port=4
  u_lqr_i_p (V) : Inport  Port=5
  u_lqr_i_y (V) : Inport  Port=6
  u_ol (V) : Inport  Port=7
  Choose Pitch Relay : MultiPortSwitch  Inputs=2
  Choose Yaw Relay : MultiPortSwitch  Inputs=2
  Constant : Constant  Value=0
  Demux1 : Demux  Outputs=2
  FF+LQR/FF+LQR+I Switch : Subsystem
  Latch: Pitch Voltage : Subsystem
  Latch: Yaw Voltage : Subsystem
  Pitch Relay : simulink/Logic and Bit Operations/Compare To Constant  relop===  const=3.0  LogicOutDataTypeMode=uint8  ZeroCross=off
  Pitch: u_ol_p +LQR : Sum
  Pitch: Add 1 : Bias  Bias=1
  Yaw Relay : simulink/Logic and Bit Operations/Compare To Constant  relop===  const=4  LogicOutDataTypeMode=uint8  ZeroCross=off
  Yaw: u_ol_y +LQR : Sum
  Yaw: Add 1 : Bias  Bias=1
  u_pitch (V) : Outport
  u_yaw (V) : Outport  Port=2
  wires:
  FF+LQR/FF+LQR+I Switch/1(u_pitch (V)) -> Latch: Pitch Voltage/2(u (V))
  FF+LQR/FF+LQR+I Switch/2(u_yaw (V)) -> Latch: Yaw Voltage/2(u (V))
  u_ff_p (V)/1 -> FF+LQR/FF+LQR+I Switch/2(u_ff_p (V))
  u_lqr_p (V)/1 -> FF+LQR/FF+LQR+I Switch/3(u_lqr_p (V))
  u_lqr_y (V)/1 -> FF+LQR/FF+LQR+I Switch/4(u_lqr_y (V))
  u_lqr_i_p (V)/1 -> FF+LQR/FF+LQR+I Switch/5(u_lqr_i_p (V))
  u_lqr_i_y (V)/1 -> FF+LQR/FF+LQR+I Switch/6(u_lqr_i_y (V))
  Latch: Pitch Voltage/1(u_latch (V)) -> Pitch: u_ol_p +LQR/2
  Latch: Yaw Voltage/1(u_latch (V)) -> Yaw: u_ol_y +LQR/2
  switch/1 -> FF+LQR/FF+LQR+I Switch/1(switch), Latch: Pitch Voltage/1(switch), Latch: Yaw Voltage/1(switch), Pitch Relay/1, Yaw Relay/1
  Pitch: u_ol_p +LQR/1 -> u_pitch (V)/1
  Yaw: u_ol_y +LQR/1 -> u_yaw (V)/1
  Pitch Relay/1 -> Pitch: Add 1/1
  Pitch: Add 1/1 -> Choose Pitch Relay/1
  u_ol (V)/1 -> Demux1/1
  Yaw Relay/1 -> Yaw: Add 1/1
  Yaw: Add 1/1 -> Choose Yaw Relay/1
  Constant/1 -> Choose Pitch Relay/2, Choose Yaw Relay/2
  Demux1/1 -> Choose Pitch Relay/3
  Demux1/2 -> Choose Yaw Relay/3
  Choose Yaw Relay/1 -> Yaw: u_ol_y +LQR/1
  Choose Pitch Relay/1 -> Pitch: u_ol_p +LQR/1

== system q_heli_2d_ff_lqr_i/Desired Position from Joystick/Convert (-1,1) to (0,1) ==
  note: Inverse input and change range from (-1,1) to (0,1)
  input : Inport
  Bias : Bias  Bias=1
  Constant : Constant  Value=2
  Divide : Product  Inputs=*/
  Inverse : Gain  Gain=-1
  output : Outport
  wires:
  Constant/1 -> Divide/2
  Bias/1 -> Divide/1
  input/1 -> Inverse/1
  Divide/1 -> output/1
  Inverse/1 -> Bias/1

== system q_heli_2d_ff_lqr_i/2 DOF Helicopter - Closed-loop Actual System/2DOF HELI: FF+LQR Controller/Pitch feed-forward controller ==
  note: Desired pitch angle
  theta_d (rad) : Inport
  Feed-forward Pitch Gain : Gain  Gain=l_cm*m_heli*g / K_pp
  Trigonometric Function : Trigonometry  Operator=cos  OutputSignalType=real
  u_ff (V) : Outport
  wires:
  Trigonometric Function/1 -> Feed-forward Pitch Gain/1
  Feed-forward Pitch Gain/1 -> u_ff (V)/1
  theta_d (rad)/1 -> Trigonometric Function/1

== system q_heli_2d_ff_lqr_i/2 DOF Helicopter - Closed-loop Actual System/2DOF HELI: FF+LQR+I Controller/Pitch Integral Antiwidup ==
  note: u
  note: v
  note: Pitch: Integral control with anti-windup.
  pitch_err (rad) : Inport
  yaw_err (rad) : Inport  Port=2
  reset : Inport  Port=3
  Integral Input  (V/s) : Sum
  Integrator : Integrator  ExternalReset=rising
  Pitch Integral Control Gain: K(1,5) : Gain  Gain=Ki(1,5)  Multiplication=Matrix(K*u)
  Pitch Reset Time : Gain  Gain=1/Tr_p
  Saturate : Saturate  UpperLimit=SAT_INT_ERR_PITCH  LowerLimit=-SAT_INT_ERR_PITCH
  Sum : Sum  Inputs=|++
  Yaw Cross-Integral Control Gain: K(1,6) : Gain  Gain=Ki(1,6)  Multiplication=Matrix(K*u)
  u-v : Sum  Inputs=-+
  u_i_pitch (V) : Outport
  wires:
  pitch_err (rad)/1 -> Pitch Integral Control Gain: K(1,5)/1
  Integrator/1 -> u-v/1, Saturate/1
  Saturate/1 -> u_i_pitch (V)/1, u-v/2
  u-v/1 -> Pitch Reset Time/1
  Sum/1 -> Integrator/1
  Pitch Reset Time/1 -> Sum/2
  reset/1 -> Integrator/2
  yaw_err (rad)/1 -> Yaw Cross-Integral Control Gain: K(1,6)/1
  Pitch Integral Control Gain: K(1,5)/1 -> Integral Input  (V/s)/1
  Yaw Cross-Integral Control Gain: K(1,6)/1 -> Integral Input  (V/s)/2
  Integral Input  (V/s)/1 -> Sum/1

== system q_heli_2d_ff_lqr_i/2 DOF Helicopter - Closed-loop Actual System/2DOF HELI: FF+LQR+I Controller/Pitch feed-forward controller ==
  note: Desired pitch angle
  theta_d (rad) : Inport
  Feed-forward Pitch Gain : Gain  Gain=l_cm*m_heli*g / K_pp
  Trigonometric Function : Trigonometry  Operator=cos  OutputSignalType=real
  u_ff (V) : Outport
  wires:
  Trigonometric Function/1 -> Feed-forward Pitch Gain/1
  Feed-forward Pitch Gain/1 -> u_ff (V)/1
  theta_d (rad)/1 -> Trigonometric Function/1

== system q_heli_2d_ff_lqr_i/2 DOF Helicopter - Closed-loop Actual System/2DOF HELI: FF+LQR+I Controller/Yaw Integral Antiwidup ==
  note: v
  note: u
  note: Yaw: Integral control with anti-windup.
  pitch_err (rad) : Inport
  yaw_err (rad) : Inport  Port=2
  reset : Inport  Port=3
  Integral Input  (V/s) : Sum
  Integrator : Integrator  ExternalReset=rising
  Pitch Cross-Integral Control Gain: K(2,5) : Gain  Gain=Ki(2,5)  Multiplication=Matrix(K*u)
  Saturate : Saturate  UpperLimit=SAT_INT_ERR_YAW  LowerLimit=-SAT_INT_ERR_YAW
  Sum : Sum  Inputs=|++
  Yaw Integral Control Gain: K(2,6) : Gain  Gain=Ki(2,6)  Multiplication=Matrix(K*u)
  Yaw Reset Time : Gain  Gain=1/Tr_y
  u-v : Sum  Inputs=-+
  u_i_yaw (V) : Outport
  wires:
  Yaw Reset Time/1 -> Sum/2
  Sum/1 -> Integrator/1
  u-v/1 -> Yaw Reset Time/1
  Saturate/1 -> u-v/2, u_i_yaw (V)/1
  Integrator/1 -> Saturate/1, u-v/1
  yaw_err (rad)/1 -> Yaw Integral Control Gain: K(2,6)/1
  reset/1 -> Integrator/2
  pitch_err (rad)/1 -> Pitch Cross-Integral Control Gain: K(2,5)/1
  Yaw Integral Control Gain: K(2,6)/1 -> Integral Input  (V/s)/1
  Pitch Cross-Integral Control Gain: K(2,5)/1 -> Integral Input  (V/s)/2
  Integral Input  (V/s)/1 -> Sum/1

== system q_heli_2d_ff_lqr_i/2 DOF Helicopter - Closed-loop Actual System/Controller Switch/FF+LQR/FF+LQR+I Switch ==
  note: Add corresponding controllers for the pitch and yaw axes of the 2DOF HELI.
  switch : Inport
  u_ff_p (V) : Inport  Port=2
  u_lqr_p (V) : Inport  Port=3
  u_lqr_y (V) : Inport  Port=4
  u_lqr_i_p (V) : Inport  Port=5
  u_lqr_i_y (V) : Inport  Port=6
  Pitch Control  Switch : MultiPortSwitch  Inputs=2
  Pitch: FF+LQR : Sum
  Yaw Control  Switch : MultiPortSwitch  Inputs=2
  u_pitch (V) : Outport
  u_yaw (V) : Outport  Port=2
  wires:
  Pitch Control  Switch/1 -> Pitch: FF+LQR/2
  u_ff_p (V)/1 -> Pitch: FF+LQR/1
  Pitch: FF+LQR/1 -> u_pitch (V)/1
  u_lqr_p (V)/1 -> Pitch Control  Switch/2
  u_lqr_y (V)/1 -> Yaw Control  Switch/2
  Yaw Control  Switch/1 -> u_yaw (V)/1
  u_lqr_i_p (V)/1 -> Pitch Control  Switch/3
  u_lqr_i_y (V)/1 -> Yaw Control  Switch/3
  switch/1 -> Pitch Control  Switch/1, Yaw Control  Switch/1

== system q_heli_2d_ff_lqr_i/2 DOF Helicopter - Closed-loop Actual System/Controller Switch/Latch: Pitch Voltage ==
  switch : Inport
  u (V) : Inport  Port=2
  Add : Sum
  Compare To Constant : simulink/Logic and Bit Operations/Compare To Constant  relop=>=  const=3.0  LogicOutDataTypeMode=uint8  ZeroCross=off
  Constant : Constant
  Memory : Memory
  Switch : MultiPortSwitch  Inputs=2
  u_latch (V) : Outport
  wires:
  Switch/1 -> Memory/1, u_latch (V)/1
  Memory/1 -> Switch/3
  Add/1 -> Switch/1
  u (V)/1 -> Switch/2
  switch/1 -> Compare To Constant/1
  Compare To Constant/1 -> Add/1
  Constant/1 -> Add/2

== system q_heli_2d_ff_lqr_i/2 DOF Helicopter - Closed-loop Actual System/Controller Switch/Latch: Yaw Voltage ==
  switch : Inport
  u (V) : Inport  Port=2
  Add : Sum
  Compare To Constant : simulink/Logic and Bit Operations/Compare To Constant  relop=>=  const=3.0  LogicOutDataTypeMode=uint8  ZeroCross=off
  Constant : Constant
  Memory : Memory
  Switch : MultiPortSwitch  Inputs=2
  u_latch (V) : Outport
  wires:
  Constant/1 -> Add/2
  Compare To Constant/1 -> Add/1
  switch/1 -> Compare To Constant/1
  u (V)/1 -> Switch/2
  Add/1 -> Switch/1
  Memory/1 -> Switch/3
  Switch/1 -> u_latch (V)/1, Memory/1

== system q_heli_2d_ff_lqr_i/2 DOF Helicopter - Closed-loop System Simulation/2DOF HELI: FF+LQR Controller/Pitch feed-forward controller ==
  note: Desired pitch angle
  theta_d (rad) : Inport
  Feed-forward Pitch Gain : Gain  Gain=l_cm*m_heli*g / K_pp
  Trigonometric Function : Trigonometry  Operator=cos  OutputSignalType=real
  u_ff (V) : Outport
  wires:
  theta_d (rad)/1 -> Trigonometric Function/1
  Feed-forward Pitch Gain/1 -> u_ff (V)/1
  Trigonometric Function/1 -> Feed-forward Pitch Gain/1

== system q_heli_2d_ff_lqr_i/2 DOF Helicopter - Closed-loop System Simulation/2DOF HELI: FF+LQR+I Controller/Pitch Integral Antiwidup ==
  note: u
  note: v
  note: Pitch: Integral control with anti-windup.
  pitch_err (rad) : Inport
  yaw_err (rad) : Inport  Port=2
  reset : Inport  Port=3
  Integral Input  (V/s) : Sum
  Integrator : Integrator  ExternalReset=rising
  Pitch Integral Control Gain: K(1,5) : Gain  Gain=Ki(1,5)  Multiplication=Matrix(K*u)
  Pitch Reset Time : Gain  Gain=1/Tr_p
  Saturate : Saturate  UpperLimit=SAT_INT_ERR_PITCH  LowerLimit=-SAT_INT_ERR_PITCH
  Sum : Sum  Inputs=|++
  Yaw Cross-Integral Control Gain: K(1,6) : Gain  Gain=Ki(1,6)  Multiplication=Matrix(K*u)
  u-v : Sum  Inputs=-+
  u_i_pitch (V) : Outport
  wires:
  pitch_err (rad)/1 -> Pitch Integral Control Gain: K(1,5)/1
  Integrator/1 -> u-v/1, Saturate/1
  Saturate/1 -> u_i_pitch (V)/1, u-v/2
  u-v/1 -> Pitch Reset Time/1
  Sum/1 -> Integrator/1
  Pitch Reset Time/1 -> Sum/2
  reset/1 -> Integrator/2
  yaw_err (rad)/1 -> Yaw Cross-Integral Control Gain: K(1,6)/1
  Pitch Integral Control Gain: K(1,5)/1 -> Integral Input  (V/s)/1
  Yaw Cross-Integral Control Gain: K(1,6)/1 -> Integral Input  (V/s)/2
  Integral Input  (V/s)/1 -> Sum/1

== system q_heli_2d_ff_lqr_i/2 DOF Helicopter - Closed-loop System Simulation/2DOF HELI: FF+LQR+I Controller/Pitch feed-forward controller ==
  note: Desired pitch angle
  theta_d (rad) : Inport
  Feed-forward Pitch Gain : Gain  Gain=l_cm*m_heli*g / K_pp
  Trigonometric Function : Trigonometry  Operator=cos  OutputSignalType=real
  u_ff (V) : Outport
  wires:
  Trigonometric Function/1 -> Feed-forward Pitch Gain/1
  Feed-forward Pitch Gain/1 -> u_ff (V)/1
  theta_d (rad)/1 -> Trigonometric Function/1

== system q_heli_2d_ff_lqr_i/2 DOF Helicopter - Closed-loop System Simulation/2DOF HELI: FF+LQR+I Controller/Yaw Integral Antiwidup ==
  note: v
  note: u
  note: Yaw: Integral control with anti-windup.
  pitch_err (rad) : Inport
  yaw_err (rad) : Inport  Port=2
  reset : Inport  Port=3
  Integral Input  (V/s) : Sum
  Integrator : Integrator  ExternalReset=rising
  Pitch Cross-Integral Control Gain: K(2,5) : Gain  Gain=Ki(2,5)  Multiplication=Matrix(K*u)
  Saturate : Saturate  UpperLimit=SAT_INT_ERR_YAW  LowerLimit=-SAT_INT_ERR_YAW
  Sum : Sum  Inputs=|++
  Yaw Integral Control Gain: K(2,6) : Gain  Gain=Ki(2,6)  Multiplication=Matrix(K*u)
  Yaw Reset Time : Gain  Gain=1/Tr_y
  u-v : Sum  Inputs=-+
  u_i_yaw (V) : Outport
  wires:
  Yaw Reset Time/1 -> Sum/2
  Sum/1 -> Integrator/1
  u-v/1 -> Yaw Reset Time/1
  Saturate/1 -> u-v/2, u_i_yaw (V)/1
  Integrator/1 -> Saturate/1, u-v/1
  yaw_err (rad)/1 -> Yaw Integral Control Gain: K(2,6)/1
  reset/1 -> Integrator/2
  pitch_err (rad)/1 -> Pitch Cross-Integral Control Gain: K(2,5)/1
  Yaw Integral Control Gain: K(2,6)/1 -> Integral Input  (V/s)/1
  Pitch Cross-Integral Control Gain: K(2,5)/1 -> Integral Input  (V/s)/2
  Integral Input  (V/s)/1 -> Sum/1

== system q_heli_2d_ff_lqr_i/2 DOF Helicopter - Closed-loop System Simulation/2DOF HELI: Nonlinear Model/Gravitational Torque ==
  theta (rad) : Inport
  Trigonometric Function : Trigonometry  Operator=cos  OutputSignalType=real
  m*g*lcm : Gain  Gain=m_heli*g*l_cm
  tau_g (N.m) : Outport
  wires:
  Trigonometric Function/1 -> m*g*lcm/1
  theta (rad)/1 -> Trigonometric Function/1
  m*g*lcm/1 -> tau_g (N.m)/1

== system q_heli_2d_ff_lqr_i/2 DOF Helicopter - Closed-loop System Simulation/2DOF HELI: Nonlinear Model/Pitch Position Dependent Torque ==
  theta (rad) : Inport
  psi_dot (rad/s) : Inport  Port=2
  Product : Product  Inputs=4  RndMeth=Zero
  cos(theta) : Trigonometry  Operator=cos  OutputSignalType=real
  m*lcm^2 : Gain  Gain=m_heli*l_cm^2
  sin(theta) : Trigonometry  OutputSignalType=real
  out (N.m) : Outport
  wires:
  m*lcm^2/1 -> out (N.m)/1
  cos(theta)/1 -> Product/2
  sin(theta)/1 -> Product/1
  Product/1 -> m*lcm^2/1
  theta (rad)/1 -> sin(theta)/1, cos(theta)/1
  psi_dot (rad/s)/1 -> Product/3, Product/4

== system q_heli_2d_ff_lqr_i/2 DOF Helicopter - Closed-loop System Simulation/2DOF HELI: Nonlinear Model/Yaw Inertia ==
  theta (rad) : Inport
  Sum3 : Sum
  Yaw Inertia : Constant  Value=J_eq_y
  cos(theta) : Trigonometry  Operator=cos  OutputSignalType=real
  cos(theta)^2 : Product  RndMeth=Zero
  m_heli*l_cm^2 : Gain  Gain=m_heli*l_cm^2
  J_y (kg.m^2) : Outport
  wires:
  cos(theta)^2/1 -> m_heli*l_cm^2/1
  Yaw Inertia/1 -> Sum3/1
  m_heli*l_cm^2/1 -> Sum3/2
  theta (rad)/1 -> cos(theta)/1
  Sum3/1 -> J_y (kg.m^2)/1
  cos(theta)/1 -> cos(theta)^2/1, cos(theta)^2/2

== system q_heli_2d_ff_lqr_i/2 DOF Helicopter - Closed-loop System Simulation/2DOF HELI: Nonlinear Model/Yaw Position Dependent Torque ==
  theta (rad) : Inport
  psi (rad) : Inport  Port=2
  theta_dot (rad/s) : Inport  Port=3
  psi_dot (rad/s) : Inport  Port=4
  2*m*lcm^2 : Gain  Gain=2*m_heli*l_cm^2
  Product : Product  Inputs=4  RndMeth=Zero
  cos(theta) : Trigonometry  Operator=cos  OutputSignalType=real
  sin(psi) : Trigonometry  OutputSignalType=real
  out (N.m) : Outport
  wires:
  psi (rad)/1 -> sin(psi)/1
  theta (rad)/1 -> cos(theta)/1
  Product/1 -> 2*m*lcm^2/1
  cos(theta)/1 -> Product/1
  sin(psi)/1 -> Product/2
  theta_dot (rad/s)/1 -> Product/3
  psi_dot (rad/s)/1 -> Product/4
  2*m*lcm^2/1 -> out (N.m)/1

== system q_heli_2d_ff_lqr_i/2 DOF Helicopter - Closed-loop System Simulation/Controller Switch/FF+LQR/FF+LQR+I Switch ==
  note: Add corresponding controllers for the pitch and yaw axes of the 2DOF HELI.
  switch : Inport
  u_ff_p (V) : Inport  Port=2
  u_lqr_p (V) : Inport  Port=3
  u_lqr_y (V) : Inport  Port=4
  u_lqr_i_p (V) : Inport  Port=5
  u_lqr_i_y (V) : Inport  Port=6
  Pitch Control  Switch : MultiPortSwitch  Inputs=2
  Pitch: FF+LQR : Sum
  Yaw Control  Switch : MultiPortSwitch  Inputs=2
  u_pitch (V) : Outport
  u_yaw (V) : Outport  Port=2
  wires:
  Pitch Control  Switch/1 -> Pitch: FF+LQR/2
  u_ff_p (V)/1 -> Pitch: FF+LQR/1
  Pitch: FF+LQR/1 -> u_pitch (V)/1
  u_lqr_p (V)/1 -> Pitch Control  Switch/2
  u_lqr_y (V)/1 -> Yaw Control  Switch/2
  Yaw Control  Switch/1 -> u_yaw (V)/1
  u_lqr_i_p (V)/1 -> Pitch Control  Switch/3
  u_lqr_i_y (V)/1 -> Yaw Control  Switch/3
  switch/1 -> Pitch Control  Switch/1, Yaw Control  Switch/1

== system q_heli_2d_ff_lqr_i/2 DOF Helicopter - Closed-loop System Simulation/Controller Switch/Latch: Pitch Voltage ==
  switch : Inport
  u (V) : Inport  Port=2
  Add : Sum
  Compare To Constant : simulink/Logic and Bit Operations/Compare To Constant  relop=>=  const=3.0  LogicOutDataTypeMode=uint8  ZeroCross=off
  Constant : Constant
  Memory : Memory
  Switch : MultiPortSwitch  Inputs=2
  u_latch (V) : Outport
  wires:
  Switch/1 -> Memory/1, u_latch (V)/1
  Memory/1 -> Switch/3
  Add/1 -> Switch/1
  u (V)/1 -> Switch/2
  switch/1 -> Compare To Constant/1
  Compare To Constant/1 -> Add/1
  Constant/1 -> Add/2

== system q_heli_2d_ff_lqr_i/2 DOF Helicopter - Closed-loop System Simulation/Controller Switch/Latch: Yaw Voltage ==
  switch : Inport
  u (V) : Inport  Port=2
  Add : Sum
  Compare To Constant : simulink/Logic and Bit Operations/Compare To Constant  relop=>=  const=3.0  LogicOutDataTypeMode=uint8  ZeroCross=off
  Constant : Constant
  Memory : Memory
  Switch : MultiPortSwitch  Inputs=2
  u_latch (V) : Outport
  wires:
  Constant/1 -> Add/2
  Compare To Constant/1 -> Add/1
  switch/1 -> Compare To Constant/1
  u (V)/1 -> Switch/2
  Add/1 -> Switch/1
  Memory/1 -> Switch/3
  Switch/1 -> u_latch (V)/1, Memory/1
